simulink model "bh_quick_step"  (R2017b)
settings: Solver=VariableStepAuto  StartTime=0.0  StopTime=10.0  RelTol=1e-3
settings Model: Creator=bhorton  LastModifiedBy=bhorton

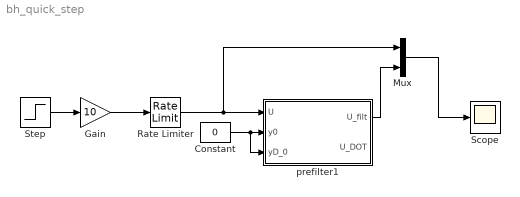
== system bh_quick_step ==
  Constant : Constant  Value=0
  Gain : Gain  Gain=10
  Mux : Mux  Inputs=2
  Rate Limiter : RateLimiter  RisingSlewLimit=5  SampleTimeMode=inherited
  Scope : Scope
  Step : Step  SampleTime=0
  prefilter1 : Subsystem  mask(Derivative Estimation){wn=2*pi*5, p=1}
      mask prompts: wn "Natural frequency, wn (rad/sec)"; p "Damping ratio, p"
      mask help:
      | A simple derivative estimator using a 2nd order representation between input and output.
      |
      | The integrators use a discrete FORWARd Euler rule, and a sample time needs to be specified.
      mask init:
      | str1 = sprintf('wn = %.2f', wn);
      | str2 = sprintf('p  = %.2f', p);
      | %str3 = sprintf('dt = %.2f', dt);
      | %str = char(str1,str2,str3);
      | %str3 = sprintf('dt = %.2f', dt);
      | str = char(str1,str2);
      mask Display: disp(str)
  wires:
  Step/1 -> Gain/1
  Mux/1 -> Scope/1
  prefilter1/1(U_filt) -> Mux/2
  Gain/1 -> Rate Limiter/1
  Rate Limiter/1 -> Mux/1, prefilter1/1(U)
  Constant/1 -> prefilter1/3(yD_0), prefilter1/2(y0)

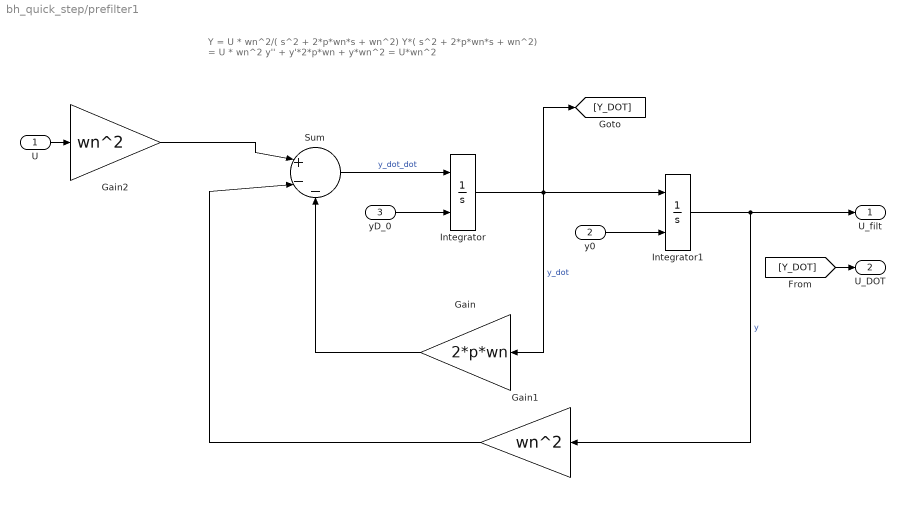
== system bh_quick_step/prefilter1 ==
  note: Y = U *     wn^2/( s^2 + 2*p*wn*s + wn^2)
      | Y*( s^2 + 2*p*wn*s + wn^2) = U * wn^2
      |
      | y'' + y'*2*p*wn + y*wn^2 = U*wn^2
  U : Inport
  y0 : Inport  Port=2
  yD_0 : Inport  Port=3
  Gain : Gain  Gain=2*p*wn
  Gain1 : Gain  Gain=wn^2
  Gain2 : Gain  Gain=wn^2
  Integrator : Integrator  InitialConditionSource=external
  Integrator1 : Integrator  InitialConditionSource=external
  Sum : Sum  Inputs=|+--
  U_filt : Outport
  U_DOT : Outport  Port=2
  wires:
  Integrator/1 -> [Y_DOT], Gain/1, Integrator1/1  "y_dot"
  Sum/1 -> Integrator/1  "y_dot_dot"
  Integrator1/1 -> Gain1/1, U_filt/1  "y"
  U/1 -> Gain2/1
  Gain2/1 -> Sum/1
  Gain/1 -> Sum/3
  Gain1/1 -> Sum/2
  [Y_DOT] -> U_DOT/1
  yD_0/1 -> Integrator/2
  y0/1 -> Integrator1/2
